simulink model "Lab2atemplatev2"  (R2014a)
settings: Solver=FixedStepDiscrete  SolverMode=SingleTasking  StartTime=0.0  StopTime=inf  FixedStep=Ts  RelTol=1e-3
values from neighbouring files (symbols this model uses):
  KdA = 1    [initScript.m]
  KdB = 1    [initScript.m]
  KdC = 1    [initScript.m]
  KiA = 5    [initScript.m]
  KiB = 5    [initScript.m]
  KiC = 5    [initScript.m]
  KpA = 100    [initScript.m]
  KpB = 100    [initScript.m]
  KpC = 100    [initScript.m]
  traj_A = q(1,1:end)    [initScript.m]
  traj_B = q(2,1:end)    [initScript.m]
  traj_C = q(3,1:end)    [initScript.m]
  traj_dA = q_dot(1,1:end)    [initScript.m]
  traj_dB = q_dot(2,1:end)    [initScript.m]
  traj_dC = q_dot(3,1:end)    [initScript.m]
  Ts_traj = .2    (= 0.2)    [initScript.m]
libraries: legonxtlib x6, cstblocks x6
settings Model: SimulationMode=external  ExtModeTrigDuration=2  Creator=pwterry  LastModifiedBy=ozmen
settings OptimizationCC: OptimizeModelRefInitCode=on  LifeSpan=1
settings DebuggingCC: UnderspecifiedInitializationDetection=Classic  SolverPrmCheckMsg=none
settings HardwareCC: ProdLargestAtomicInteger=Long  ProdLargestAtomicFloat=Float  ProdEndianess=LittleEndian  ProdHWDeviceType=ARM Compatible->ARM 7
settings RTWCC: SystemTargetFile=realtime.tlc  GenerateMakefile=off  TemplateMakefile=realtime.tmf  Description=Run on Target Hardware  RTWVerbose=off  ProcessScript=realtime_make_rtw_hook
settings STFCustomTargetCC: TargetLibSuffix=.a  GenerateSampleERTMain=on  ConcurrentExecutionCompliant=off  GeneratePreprocessorConditionals=Use local settings  ERTCustomFileBanners=on  SupportNonInlinedSFcns=off  SupportVariableSizeSignals=on  MATLABClassNameForMDSCustomization=Simulink.SoftwareTarget.ERTCustomization  GRTInterface=off  SystemTargetFile=realtime.tlc
settings ERTTargetCC: CombineOutputUpdateFcns=off  SupportContinuousTime=on  SupportVariableSizeSignals=on  ExtMode=on  ExtModeTransport=2  ExtModeMexFile=ext_serial_win32_comm_no_acks_rtt  ExtModeMexArgs=0 89 9600 30  ERTSrcFileBannerTemplate=realtime_code_template.cgt  ERTHdrFileBannerTemplate=realtime_code_template.cgt  ERTDataSrcFileTemplate=realtime_code_template.cgt  ERTDataHdrFileTemplate=realtime_code_template.cgt  ERTCustomFileTemplate=realtime_file_process.tlc

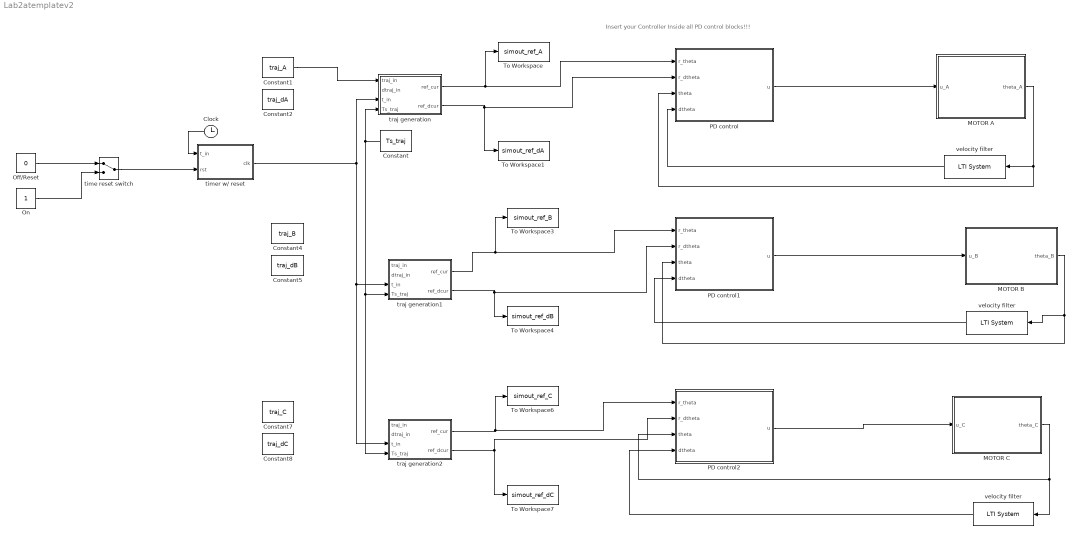
== system Lab2atemplatev2 ==
  note: Insert your Controller Inside all PD control blocks!!!
  Clock : Clock
  Constant : Constant  Value=Ts_traj
  Constant1 : Constant  Value=traj_A
  Constant2 : Constant  Value=traj_dA
  Constant4 : Constant  Value=traj_B
  Constant5 : Constant  Value=traj_dB
  Constant7 : Constant  Value=traj_C
  Constant8 : Constant  Value=traj_dC
  MOTOR A : Subsystem
  MOTOR B : Subsystem
  MOTOR C : Subsystem
  Off/Reset : Constant  Value=0
  On : Constant
  PD control : Subsystem
  PD control1 : Subsystem
  PD control2 : Subsystem
  To Workspace : ToWorkspace  VariableName=simout_ref_A  SaveFormat=Structure With Time  SampleTime=-1
  To Workspace1 : ToWorkspace  VariableName=simout_ref_dA  SaveFormat=Structure With Time  SampleTime=-1
  To Workspace3 : ToWorkspace  VariableName=simout_ref_B  SaveFormat=Structure With Time  SampleTime=-1
  To Workspace4 : ToWorkspace  VariableName=simout_ref_dB  SaveFormat=Structure With Time  SampleTime=-1
  To Workspace6 : ToWorkspace  VariableName=simout_ref_C  SaveFormat=Structure With Time  SampleTime=-1
  To Workspace7 : ToWorkspace  VariableName=simout_ref_dC  SaveFormat=Structure With Time  SampleTime=-1
  time reset switch : ManualSwitch
  timer w/ reset : MATLAB Function  TreatAsAtomicUnit=on
  traj generation : MATLAB Function  TreatAsAtomicUnit=on
  traj generation1 : MATLAB Function  TreatAsAtomicUnit=on
  traj generation2 : MATLAB Function  TreatAsAtomicUnit=on
  velocity filter : cstblocks/LTI System  sys=dttf  IC=[]
  "velocity filter  " : cstblocks/LTI System  sys=dttf  IC=[]
  "velocity filter     " : cstblocks/LTI System  sys=dttf  IC=[]
  wires:
  Constant/1 -> traj generation2/4(Ts_traj), traj generation1/4(Ts_traj), traj generation/4(Ts_traj)
  timer w/ reset/1(clk) -> traj generation1/3(t_in), traj generation2/3(t_in), traj generation/3(t_in)
  traj generation/1(ref_cur) -> PD control/1(r_theta), To Workspace/1
  traj generation/2(ref_dcur) -> PD control/2(r_dtheta), To Workspace1/1
  traj generation1/1(ref_cur) -> PD control1/1(r_theta), To Workspace3/1
  traj generation1/2(ref_dcur) -> PD control1/2(r_dtheta), To Workspace4/1
  traj generation2/1(ref_cur) -> PD control2/1(r_theta), To Workspace6/1
  traj generation2/2(ref_dcur) -> To Workspace7/1, PD control2/2(r_dtheta)
  MOTOR A/1(theta_A) -> PD control/3(theta), velocity filter/1
  MOTOR B/1(theta_B) -> PD control1/3(theta), "velocity filter  "/1
  MOTOR C/1(theta_C) -> PD control2/3(theta), "velocity filter     "/1
  Off/Reset/1 -> time reset switch/1
  On/1 -> time reset switch/2
  time reset switch/1 -> timer w/ reset/2(rst)
  Clock/1 -> timer w/ reset/1(t_in)
  "velocity filter     "/1 -> PD control2/4(dtheta)
  PD control2/1(u) -> MOTOR C/1(u_C)
  PD control1/1(u) -> MOTOR B/1(u_B)
  PD control/1(u) -> MOTOR A/1(u_A)
  velocity filter/1 -> PD control/4(dtheta)
  "velocity filter  "/1 -> PD control1/4(dtheta)
  Constant1/1 -> traj generation/1(traj_in)

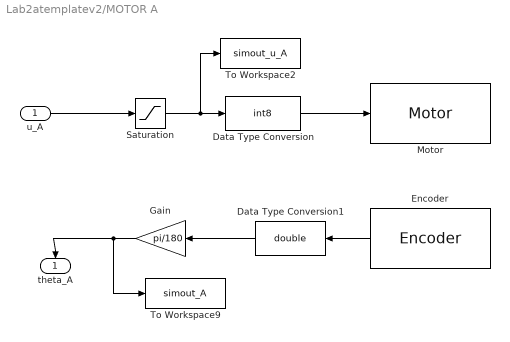
== system Lab2atemplatev2/MOTOR A ==
  u_A : Inport
  Data Type Conversion : DataTypeConversion  OutDataTypeStr=int8
  Data Type Conversion1 : DataTypeConversion  OutDataTypeStr=double
  Encoder : legonxtlib/Encoder  portNumber=A  opMode=No reset  sampleTime=Ts
  Gain : Gain  Gain=pi/180
  Motor : legonxtlib/Motor  sportNumber=A  sstopAction=Brake
  Saturation : Saturate  UpperLimit=100  LowerLimit=-100
  To Workspace2 : ToWorkspace  VariableName=simout_u_A  SaveFormat=Structure With Time  SampleTime=-1
  To Workspace9 : ToWorkspace  VariableName=simout_A  SaveFormat=Structure With Time  SampleTime=-1
  theta_A : Outport
  wires:
  u_A/1 -> Saturation/1
  Data Type Conversion1/1 -> Gain/1
  Saturation/1 -> To Workspace2/1, Data Type Conversion/1
  Encoder/1 -> Data Type Conversion1/1
  Data Type Conversion/1 -> Motor/1
  Gain/1 -> theta_A/1, To Workspace9/1

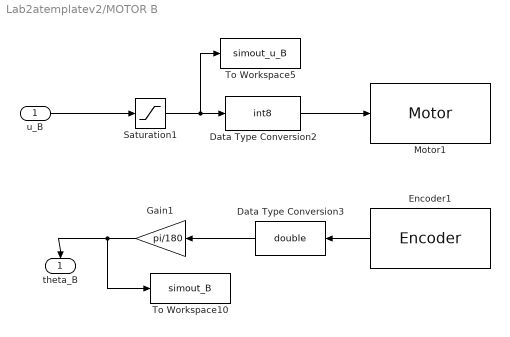
== system Lab2atemplatev2/MOTOR B ==
  u_B : Inport
  Data Type Conversion2 : DataTypeConversion  OutDataTypeStr=int8
  Data Type Conversion3 : DataTypeConversion  OutDataTypeStr=double
  Encoder1 : legonxtlib/Encoder  portNumber=B  opMode=No reset  sampleTime=Ts
  Gain1 : Gain  Gain=pi/180
  Motor1 : legonxtlib/Motor  sportNumber=B  sstopAction=Brake
  Saturation1 : Saturate  UpperLimit=100  LowerLimit=-100
  To Workspace10 : ToWorkspace  VariableName=simout_B  SaveFormat=Structure With Time  SampleTime=-1
  To Workspace5 : ToWorkspace  VariableName=simout_u_B  SaveFormat=Structure With Time  SampleTime=-1
  theta_B : Outport
  wires:
  Encoder1/1 -> Data Type Conversion3/1
  u_B/1 -> Saturation1/1
  Saturation1/1 -> To Workspace5/1, Data Type Conversion2/1
  Data Type Conversion3/1 -> Gain1/1
  Data Type Conversion2/1 -> Motor1/1
  Gain1/1 -> theta_B/1, To Workspace10/1

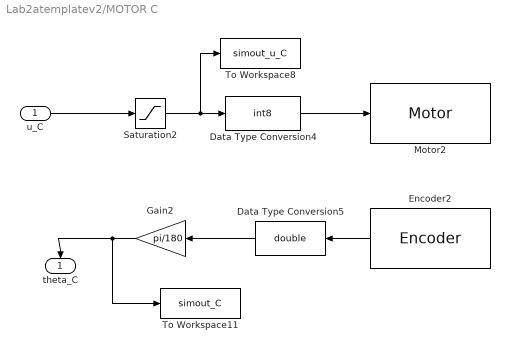
== system Lab2atemplatev2/MOTOR C ==
  u_C : Inport
  Data Type Conversion4 : DataTypeConversion  OutDataTypeStr=int8
  Data Type Conversion5 : DataTypeConversion  OutDataTypeStr=double
  Encoder2 : legonxtlib/Encoder  portNumber=C  opMode=No reset  sampleTime=Ts
  Gain2 : Gain  Gain=pi/180
  Motor2 : legonxtlib/Motor  sportNumber=C  sstopAction=Brake
  Saturation2 : Saturate  UpperLimit=100  LowerLimit=-100
  To Workspace11 : ToWorkspace  VariableName=simout_C  SaveFormat=Structure With Time  SampleTime=-1
  To Workspace8 : ToWorkspace  VariableName=simout_u_C  SaveFormat=Structure With Time  SampleTime=-1
  theta_C : Outport
  wires:
  Encoder2/1 -> Data Type Conversion5/1
  Data Type Conversion4/1 -> Motor2/1
  Data Type Conversion5/1 -> Gain2/1
  Gain2/1 -> theta_C/1, To Workspace11/1
  Saturation2/1 -> To Workspace8/1, Data Type Conversion4/1
  u_C/1 -> Saturation2/1

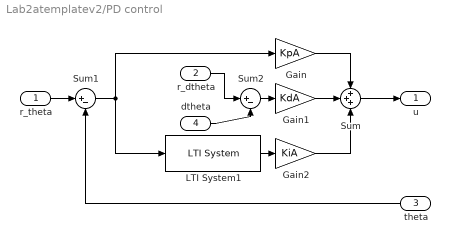
== system Lab2atemplatev2/PD control ==
  r_theta : Inport
  r_dtheta : Inport  Port=2
  theta : Inport  Port=3
  dtheta : Inport  Port=4
  Gain : Gain  Gain=KpA
  Gain1 : Gain  Gain=KdA
  Gain2 : Gain  Gain=KiA
  LTI System1 : cstblocks/LTI System  sys=itf  IC=[]
  Sum : Sum  Inputs=+++
  Sum1 : Sum  Inputs=|+-
  Sum2 : Sum  Inputs=|+-
  u : Outport
  wires:
  r_theta/1 -> Sum1/1
  theta/1 -> Sum1/2
  Sum1/1 -> LTI System1/1, Gain/1
  Gain/1 -> Sum/1
  Sum2/1 -> Gain1/1
  Gain1/1 -> Sum/2
  Sum/1 -> u/1
  LTI System1/1 -> Gain2/1
  Gain2/1 -> Sum/3
  r_dtheta/1 -> Sum2/1
  dtheta/1 -> Sum2/2

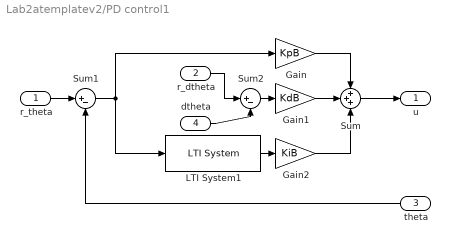
== system Lab2atemplatev2/PD control1 ==
  r_theta : Inport
  r_dtheta : Inport  Port=2
  theta : Inport  Port=3
  dtheta : Inport  Port=4
  Gain : Gain  Gain=KpB
  Gain1 : Gain  Gain=KdB
  Gain2 : Gain  Gain=KiB
  LTI System1 : cstblocks/LTI System  sys=itf  IC=[]
  Sum : Sum  Inputs=+++
  Sum1 : Sum  Inputs=|+-
  Sum2 : Sum  Inputs=|+-
  u : Outport
  wires:
  r_theta/1 -> Sum1/1
  theta/1 -> Sum1/2
  Sum1/1 -> LTI System1/1, Gain/1
  Gain/1 -> Sum/1
  Sum2/1 -> Gain1/1
  Gain1/1 -> Sum/2
  Sum/1 -> u/1
  LTI System1/1 -> Gain2/1
  Gain2/1 -> Sum/3
  r_dtheta/1 -> Sum2/1
  dtheta/1 -> Sum2/2

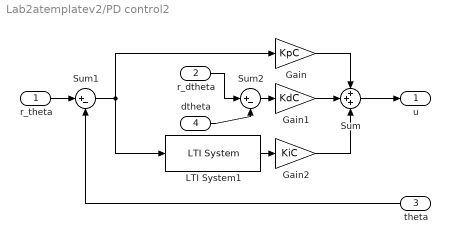
== system Lab2atemplatev2/PD control2 ==
  r_theta : Inport
  r_dtheta : Inport  Port=2
  theta : Inport  Port=3
  dtheta : Inport  Port=4
  Gain : Gain  Gain=KpC
  Gain1 : Gain  Gain=KdC
  Gain2 : Gain  Gain=KiC
  LTI System1 : cstblocks/LTI System  sys=itf  IC=[]
  Sum : Sum  Inputs=+++
  Sum1 : Sum  Inputs=|+-
  Sum2 : Sum  Inputs=|+-
  u : Outport
  wires:
  r_theta/1 -> Sum1/1
  theta/1 -> Sum1/2
  Sum1/1 -> LTI System1/1, Gain/1
  Gain/1 -> Sum/1
  Sum2/1 -> Gain1/1
  Gain1/1 -> Sum/2
  Sum/1 -> u/1
  LTI System1/1 -> Gain2/1
  Gain2/1 -> Sum/3
  r_dtheta/1 -> Sum2/1
  dtheta/1 -> Sum2/2

== matlab function Lab2atemplatev2/traj generation1 ==
  data: traj_in input; dtraj_in input; ref_cur output; t_in input; Ts_traj input; ref_dcur output
function [ref_cur, ref_dcur] = fcn(traj_in, dtraj_in, t_in, Ts_traj)
t_offset = 1;   %amt of seconds to wait before starting traj

base_numPts_per_sec = length(traj_in)/(Ts_traj*length(traj_in));
scaleFactor = 1; %Time scaling factor (# of trajectory points per second multiplier)
%Tweaking this will speed-up or slow-down the playback of traj, allowing
%for some control over resolution.
scaling = scaleFactor*base_numPts_per_sec; 
t_cur = t_in-t_offset;
time = max(t_cur,0);
%Compute the current index in the trajectory array
index_fraction = scaling*time + 1;
index = floor(index_fraction);
frac_add = index_fraction - index; % additional amount "beyond" index
%Extract the current position from the trajectory (plus interp)
if (index < length(traj_in))
    
    theta_out = (1-frac_add)*double(traj_in(index)) + ...
        frac_add*double(traj_in(index+1));
    
    dtheta_out = (1-frac_add)*double(dtraj_in(index)) + ...
        frac_add*double(dtraj_in(index+1));
    
else %If we run out of data, continue outputting the last value
    theta_out = double(traj_in(length(traj_in)));
    dtheta_out = double(dtraj_in(length(dtraj_in)));
end
ref_cur = theta_out;
ref_dcur = dtheta_out;




end

== matlab function Lab2atemplatev2/traj generation2 ==
  data: traj_in input; dtraj_in input; ref_cur output; t_in input; Ts_traj input; ref_dcur output
function [ref_cur, ref_dcur] = fcn(traj_in, dtraj_in, t_in, Ts_traj)
t_offset = 1;   %amt of seconds to wait before starting traj

base_numPts_per_sec = length(traj_in)/(Ts_traj*length(traj_in));
scaleFactor = 1; %Time scaling factor (# of trajectory points per second multiplier)
%Tweaking this will speed-up or slow-down the playback of traj, allowing
%for some control over resolution.
scaling = scaleFactor*base_numPts_per_sec; 
t_cur = t_in-t_offset;
time = max(t_cur,0);
%Compute the current index in the trajectory array
index_fraction = scaling*time + 1;
index = floor(index_fraction);
frac_add = index_fraction - index; % additional amount "beyond" index
%Extract the current position from the trajectory (plus interp)
if (index < length(traj_in))
    
    theta_out = (1-frac_add)*double(traj_in(index)) + ...
        frac_add*double(traj_in(index+1));
    
    dtheta_out = (1-frac_add)*double(dtraj_in(index)) + ...
        frac_add*double(dtraj_in(index+1));
    
else %If we run out of data, continue outputting the last value
    theta_out = double(traj_in(length(traj_in)));
    dtheta_out = double(dtraj_in(length(dtraj_in)));
end
ref_cur = theta_out;
ref_dcur = dtheta_out;




end

== matlab function Lab2atemplatev2/timer w// reset ==
  data: t_in input; clk output; rst input
function clk = fcn(t_in, rst)
persistent t_off last_rst
if isempty(t_off)
    t_off = 0;
end
if isempty(last_rst)
    last_rst = 0;
end

%if rest switch was pressed, use current time as t_offset
if abs(rst - last_rst) ~= 0
   t_off = t_in;    
end

if rst == 0
    clk = 0;    %force time to wait if reset is on
else
    clk = t_in - t_off; %output clock
end
last_rst = rst;     %update reset var

== matlab function Lab2atemplatev2/traj generation ==
  data: traj_in input; dtraj_in input; ref_cur output; t_in input; Ts_traj input; ref_dcur output
function [ref_cur, ref_dcur] = fcn(traj_in, dtraj_in, t_in, Ts_traj)
t_offset = 1;   %amt of seconds to wait before starting traj

base_numPts_per_sec = length(traj_in)/(Ts_traj*length(traj_in));
scaleFactor = 1; %Time scaling factor (# of trajectory points per second multiplier)
%Tweaking this will speed-up or slow-down the playback of traj, allowing
%for some control over resolution.
scaling = scaleFactor*base_numPts_per_sec; 
t_cur = t_in-t_offset;
time = max(t_cur,0);
%Compute the current index in the trajectory array
index_fraction = scaling*time + 1;
index = floor(index_fraction);
frac_add = index_fraction - index; % additional amount "beyond" index
%Extract the current position from the trajectory (plus interp)
if (index < length(traj_in))
    
    theta_out = (1-frac_add)*double(traj_in(index)) + ...
        frac_add*double(traj_in(index+1));
    
    dtheta_out = (1-frac_add)*double(dtraj_in(index)) + ...
        frac_add*double(dtraj_in(index+1));
    
else %If we run out of data, continue outputting the last value
    theta_out = double(traj_in(length(traj_in)));
    dtheta_out = double(dtraj_in(length(dtraj_in)));
end
ref_cur = theta_out;
ref_dcur = dtheta_out;




end
